simulink model "AFDNFSmodelMPA"  (Simulink 8.8)
settings: Solver=ode45  StartTime=0.0  StopTime=100  FixedStep=1e-3  RelTol=1e-6  EnableMultiTasking=on
InitFcn:
  | run('Methods/AFDSimInit')
  | load('SampleDatcomData.mat')
values from neighbouring files (symbols this model uses):
  nfs = TransferFunction('Plot','true')    [Main.m]    (also in NFSDatabase.sldd = SI
                Imperial
                28184.4409185639)
undefined symbols (not defined in the file or in its folder): datcom, desired, K_lat, K_long, Kobsvlat, Kobsvlong, lat, latsys, long, longsys, Newton, Raphson, sigbuilder_block
libraries: aerolibutil x13, aerolibtransform2 x1, aerolibasang x1
(part 1 of 3)
settings Model: Creator=AHKh PC  LastModifiedBy=AHKh
settings SolverCC: ZeroCrossAlgorithm=Adaptive  AutoInsertRateTranBlk=on
settings DataIOCC: LimitDataPoints=off  SaveOutput=off
settings OptimizationCC: ExpressionDepthLimit=2147483647
settings DebuggingCC: SolverPrmCheckMsg=warning
settings GRTTargetCC: CombineOutputUpdateFcns=on  GRTInterface=off

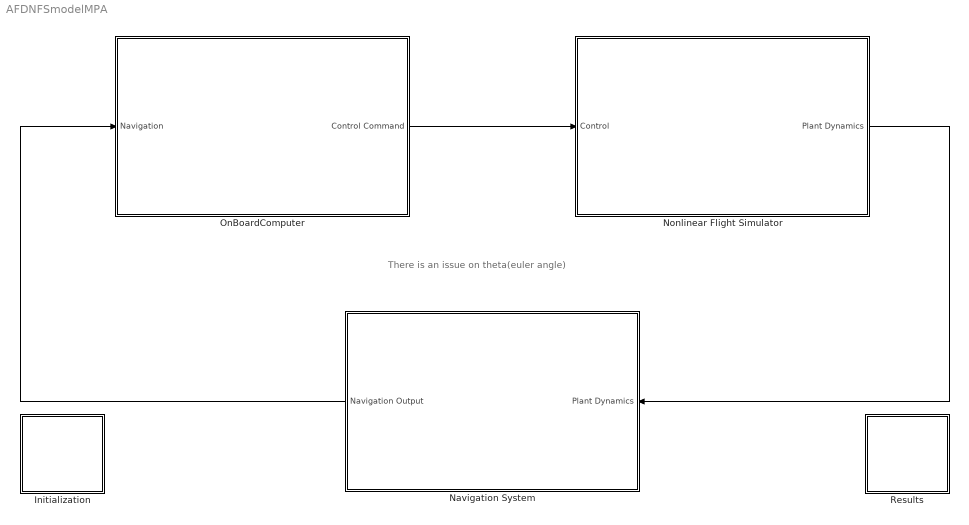
== system AFDNFSmodelMPA ==
  note: There is an issue on theta(euler angle)
  Initialization : Subsystem
      settings: OpenFcn=|
      | % edit('Methods/AFDSimInit.m')
      | !NFSData/NFS Data.xlsx
      mask Display: image(imread('iData/Initialization'))
  Navigation System : Subsystem
      mask Display: image(imread('iData/NavigationSystem'))
  Nonlinear Flight Simulator : Subsystem
      mask Display: image(imread('iData/LockheedMartinVARIOUS'));
  OnBoardComputer : Subsystem
      mask Display: image(imread('iData/OnBoardComputerESAPathfinder'));
  Results : Subsystem
      settings: OpenFcn=|
      | cd 'Methods';
      | Plotter(ned_position,euler_angles,control_commands,tout)
      | cd ..
      mask Display: image(imread('iData/Initialization'))
  wires:
  OnBoardComputer/1(Control Command) -> Nonlinear Flight Simulator/1(Control)
  Navigation System/1(Navigation Output) -> OnBoardComputer/1(Navigation)
  Nonlinear Flight Simulator/1(Plant Dynamics) -> Navigation System/1(Plant Dynamics)

== system AFDNFSmodelMPA/Initialization ==

== system AFDNFSmodelMPA/Navigation System ==
  Plant Dynamics : Inport
  Navigation Output : Outport
  wires:
  Plant Dynamics/1 -> Navigation Output/1

== system AFDNFSmodelMPA/Nonlinear Flight Simulator ==
  Control : Inport
  6DoF Nonlinear Flight Equations of Motion (Rigid Body) : Subsystem
  Forces&Moments : Subsystem
  Ground1 : Ground
  Initialization : Subsystem
  Mux : Mux  Inputs=7
  Plot : Subsystem
  Scope : Scope
  Scope1 : Scope
  Scope4 : Scope
  Plant Dynamics : Outport
  wires:
  Forces&Moments/1(Forces (Body)) -> 6DoF Nonlinear Flight Equations of Motion (Rigid Body)/1(Forces (F) (Body)), Scope1/1
  Forces&Moments/2(Moments (Body)) -> Scope4/1, 6DoF Nonlinear Flight Equations of Motion (Rigid Body)/2(Moments (M) (Body))
  6DoF Nonlinear Flight Equations of Motion (Rigid Body)/1(Linear Velocity (Body)) -> Forces&Moments/1(Linear Velocity), Plot/1(Linear Velocity (Body)), Mux/1
  Initialization/3(Initial Inertia tensor) -> 6DoF Nonlinear Flight Equations of Motion (Rigid Body)/5(Inertia Tensor (I))
  Initialization/4(Inertia tensor Change Rate) -> 6DoF Nonlinear Flight Equations of Motion (Rigid Body)/6(Inertia Tensor Change Rate (Idot))
  Control/1 -> Forces&Moments/3(Control)
  Initialization/2(Mass Consumption Rate) -> 6DoF Nonlinear Flight Equations of Motion (Rigid Body)/4(Mass Consumption Rate)
  Initialization/1(Initial Mass) -> 6DoF Nonlinear Flight Equations of Motion (Rigid Body)/3(Initial Mass)
  Initialization/5(Initial Linear Velocity Vector) -> 6DoF Nonlinear Flight Equations of Motion (Rigid Body)/7(Initial Linear  Velocity Vector)
  Initialization/6(Initial Angular Velocity Vector) -> 6DoF Nonlinear Flight Equations of Motion (Rigid Body)/8(Initial Angular  Velocity Vector)
  Initialization/7(Initial Euler Angles) -> 6DoF Nonlinear Flight Equations of Motion (Rigid Body)/9(Initial Euler Angles)
  6DoF Nonlinear Flight Equations of Motion (Rigid Body)/2(Angular Velocity (Body)) -> Forces&Moments/2(Angular Velocity), Plot/2(Angular Velocity (Body)), Mux/2
  6DoF Nonlinear Flight Equations of Motion (Rigid Body)/4(Angular Acceleration (Body)) -> Plot/4(Angular Acceleration (Body)), Mux/4
  Initialization/8(Initial Location (NED)) -> 6DoF Nonlinear Flight Equations of Motion (Rigid Body)/10(Initial Location (NED))
  6DoF Nonlinear Flight Equations of Motion (Rigid Body)/3(Linear Acceleration (Body)) -> Plot/3(Linear Acceleration (Body)), Mux/3
  6DoF Nonlinear Flight Equations of Motion (Rigid Body)/7(Velocity (NED)) -> Plot/7(Velocity (NED)), Mux/7
  Ground1/1 -> Scope/1
  6DoF Nonlinear Flight Equations of Motion (Rigid Body)/6(Position (NED)) -> Forces&Moments/5(Position), Plot/6(Position (NED)), Mux/6
  6DoF Nonlinear Flight Equations of Motion (Rigid Body)/5(Euler Angles) -> Forces&Moments/4(Attitute), Plot/5(Euler Angles), Mux/5
  Mux/1 -> Plant Dynamics/1

== system AFDNFSmodelMPA/OnBoardComputer ==
  Navigation : Inport
  Control System : Subsystem
  Guidance Algorithm : Subsystem
  Control Command : Outport
  wires:
  Navigation/1 -> Guidance Algorithm/1(Navigation)
  Guidance Algorithm/1(Navigation data & Guidance Command) -> Control System/1(Guidance Command)
  Control System/1(Control Command) -> Control Command/1

== system AFDNFSmodelMPA/Results ==

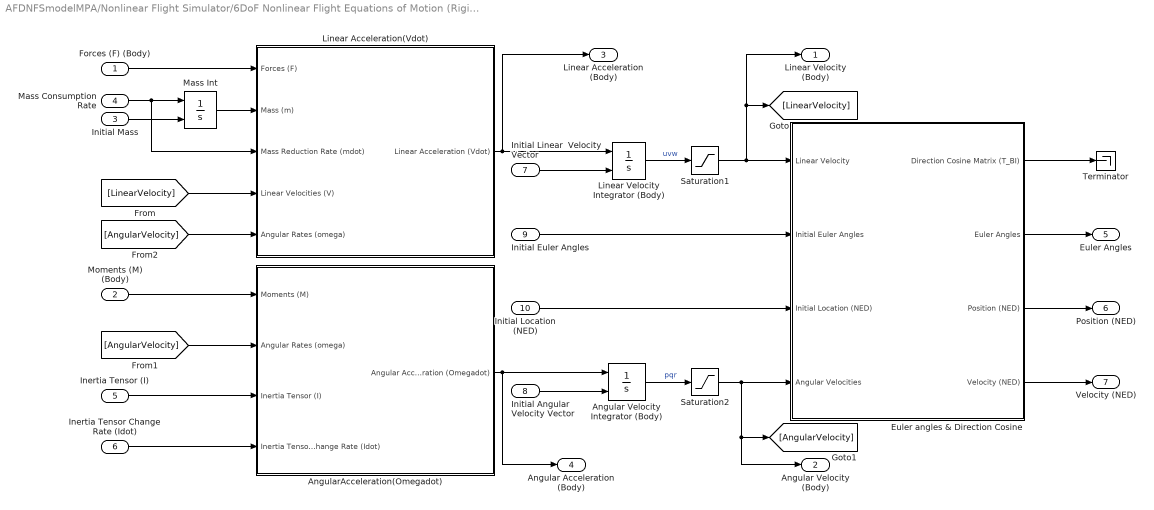
== system AFDNFSmodelMPA/Nonlinear Flight Simulator/6DoF Nonlinear Flight Equations of Motion (Rigid Body) ==
  Forces (F) (Body) : Inport
  Moments (M) (Body) : Inport  Port=2  PortDimensions=[3,1]
  Initial Mass : Inport  Port=3
  Mass Consumption Rate : Inport  Port=4
  Inertia Tensor (I) : Inport  Port=5
  Inertia Tensor Change Rate (Idot) : Inport  Port=6
  Initial Linear  Velocity Vector : Inport  Port=7
  Initial Angular  Velocity Vector : Inport  Port=8
  Initial Euler Angles : Inport  Port=9
  Initial Location (NED) : Inport  Port=10
  Angular Velocity Integrator (Body) : Integrator  InitialConditionSource=external  InitialCondition=nfs.angularvel0
  AngularAcceleration(Omegadot) : Subsystem
  Euler angles & Direction Cosine : Subsystem
  Linear Acceleration(Vdot) : Subsystem
  Linear Velocity Integrator (Body) : Integrator  InitialConditionSource=external  InitialCondition=nfs.crusevelvec  ContinuousStateAttributes='BodyVelocity'
  Mass Int : Integrator  InitialConditionSource=external  InitialCondition=nfs.crusevelvec  ContinuousStateAttributes='BodyVelocity'
  Saturation1 : Saturate  UpperLimit=500  LowerLimit=-500
  Saturation2 : Saturate  UpperLimit=500  LowerLimit=-500
  Terminator : Terminator
  Linear Velocity (Body) : Outport
  Angular Velocity (Body) : Outport  Port=2
  Linear Acceleration (Body) : Outport  Port=3
  Angular Acceleration (Body) : Outport  Port=4
  Euler Angles : Outport  Port=5
  Position (NED) : Outport  Port=6
  Velocity (NED) : Outport  Port=7
  wires:
  Initial Mass/1 -> Mass Int/2
  Mass Int/1 -> Linear Acceleration(Vdot)/2(Mass (m))
  Mass Consumption Rate/1 -> Linear Acceleration(Vdot)/3(Mass Reduction Rate (mdot)), Mass Int/1
  Linear Velocity Integrator (Body)/1 -> Saturation1/1  "uvw"
  Angular Velocity Integrator (Body)/1 -> Saturation2/1  "pqr"
  Inertia Tensor (I)/1 -> AngularAcceleration(Omegadot)/3(Inertia Tensor (I))
  Inertia Tensor Change Rate (Idot)/1 -> AngularAcceleration(Omegadot)/4(Inertia Tensor Change Rate (Idot))
  Euler angles & Direction Cosine/1(Direction Cosine Matrix (T_BI)) -> Terminator/1
  Initial Location (NED)/1 -> Euler angles & Direction Cosine/3(Initial Location (NED))
  Forces (F) (Body)/1 -> Linear Acceleration(Vdot)/1(Forces (F))
  Linear Acceleration(Vdot)/1(Linear Acceleration (Vdot)) -> Linear Acceleration (Body)/1, Linear Velocity Integrator (Body)/1
  Initial Linear  Velocity Vector/1 -> Linear Velocity Integrator (Body)/2
  Initial Angular  Velocity Vector/1 -> Angular Velocity Integrator (Body)/2
  AngularAcceleration(Omegadot)/1(Angular Acceleration (Omegadot)) -> Angular Velocity Integrator (Body)/1, Angular Acceleration (Body)/1
  [LinearVelocity] -> Linear Acceleration(Vdot)/4(Linear Velocities (V))
  [AngularVelocity] -> Linear Acceleration(Vdot)/5(Angular Rates (omega))
  Moments (M) (Body)/1 -> AngularAcceleration(Omegadot)/1(Moments (M))
  [AngularVelocity] -> AngularAcceleration(Omegadot)/2(Angular Rates (omega))
  Initial Euler Angles/1 -> Euler angles & Direction Cosine/2(Initial Euler Angles)
  Euler angles & Direction Cosine/4(Velocity (NED)) -> Velocity (NED)/1
  Euler angles & Direction Cosine/2(Euler Angles) -> Euler Angles/1
  Euler angles & Direction Cosine/3(Position (NED)) -> Position (NED)/1
  Saturation1/1 -> Linear Velocity (Body)/1, [LinearVelocity], Euler angles & Direction Cosine/1(Linear Velocity)
  Saturation2/1 -> Angular Velocity (Body)/1, [AngularVelocity], Euler angles & Direction Cosine/4(Angular Velocities)

== system AFDNFSmodelMPA/Nonlinear Flight Simulator/Forces&Moments ==
  Linear Velocity : Inport
  Angular Velocity : Inport  Port=2  Unit=rad/s  PortDimensions=[3,1]
  Control : Inport  Port=3
  Attitute : Inport  Port=4  PortDimensions=[3,1]
  Position : Inport  Port=5
  Aero Attributes : Subsystem
  Bus Selector : BusSelector  OutputSignals=delta_f,delta_e,delta_a
  C.G Loc : Constant  Value=[0 0 0]'
  Digital DATCOM v1.0.2 : Subsystem  mask(DATCOM Aerodynamic Forces and Moments Estimation){datcom=datcom}
      mask prompts: datcom "Datcom Structure"
      mask Display:
      | port_label('input',1,'\alpha (rad)','texmode','on');
      | port_label('input',2,'\beta (rad)','texmode','on');
      | port_label('input',3,'Mach','texmode','on');
      | port_label('input',4,'h (m)','texmode','on');
      | port_label('input',5,'q_{bar}','texmode','on');
      | port_label('input',6,'d\alpha/dt (rad/s)','texmode','on');
      | port_label('input',7,'V_{body} m/s','texmode','on');
      | port_label('input',8,'\omega (rad/s)','texmode','on');
      | port_label('input',9,'\delta_F (rad)','texmode','on');
      | port_label('input',10,'\delta_E (rad)','texmode','on');
      | port_label('input',11,'\delta_A (rad)','texmode','on');
      | port_label('input',12,'C.G. (m)','texmode','on');
      | port_label('output',1,'F_{body} (N)','texmode','on');
      | port_label('output',2,'M_{body} (N.m)','texmode','on');
  HeightInENU : Gain  Gain=-1  SaturateOnIntegerOverflow=on  OutDataTypeStr=Inherit: Same as input  ParamDataTypeStr=Inherit: Same as input
  HeightInENU1 : Gain  Gain=-1  SaturateOnIntegerOverflow=on  OutDataTypeStr=Inherit: Same as input  ParamDataTypeStr=Inherit: Same as input
  Linear Velocity 1 : InportShadow
  Position 1 : InportShadow  Port=5
  Selector : Selector  InputPortWidth=3  IndexOptions=Index vector (dialog)  Indices=[3]  OutputSizes=1
  Selector1 : Selector  InputPortWidth=3  IndexOptions=Index vector (dialog)  Indices=[3]  OutputSizes=1
  Sum : Sum  Inputs=+++
  Sum1 : Sum  Inputs=+++
  Terminator1 : Terminator
  Thrust : Subsystem
  Weight : Subsystem
  Forces (Body) : Outport
  Moments (Body) : Outport  Port=2
  wires:
  HeightInENU/1 -> Aero Attributes/2(Altitude)
  Linear Velocity/1 -> Aero Attributes/1(Linear Velocity (Body))
  Aero Attributes/4(Betadot) -> Terminator1/1
  Angular Velocity/1 -> Digital DATCOM v1.0.2/8(p,q,r)
  Selector/1 -> HeightInENU1/1
  Position/1 -> Selector/1
  Position 1/1 -> Selector1/1
  HeightInENU1/1 -> Digital DATCOM v1.0.2/4(altitude)
  Selector1/1 -> HeightInENU/1
  Control/1 -> Bus Selector/1
  Bus Selector/1 -> Digital DATCOM v1.0.2/9(delta_f)  "<delta_f>"
  Bus Selector/2 -> Digital DATCOM v1.0.2/10(delta_e)  "<delta_e>"
  Bus Selector/3 -> Digital DATCOM v1.0.2/11(delta_a)  "<delta_a>"
  Linear Velocity 1/1 -> Digital DATCOM v1.0.2/7(V)
  Aero Attributes/1(Alpha) -> Digital DATCOM v1.0.2/1(alp ha)
  Aero Attributes/2(Beta) -> Digital DATCOM v1.0.2/2(beta)
  Aero Attributes/5(Dynamic Pressure) -> Digital DATCOM v1.0.2/5(qbar)
  Aero Attributes/3(Mach) -> Digital DATCOM v1.0.2/3(Mach)
  Aero Attributes/6(Alphadot) -> Digital DATCOM v1.0.2/6(alpha_dot)
  Attitute/1 -> Weight/1(Attitute)
  Digital DATCOM v1.0.2/1(F) -> Sum/1
  Weight/1(Force) -> Sum/2
  Thrust/1(Force) -> Sum/3
  Sum/1 -> Forces (Body)/1
  Weight/2(Moment) -> Sum1/2
  Digital DATCOM v1.0.2/2(M) -> Sum1/1
  Thrust/2(Moment) -> Sum1/3
  Sum1/1 -> Moments (Body)/1
  C.G Loc/1 -> Digital DATCOM v1.0.2/12(C.G.)

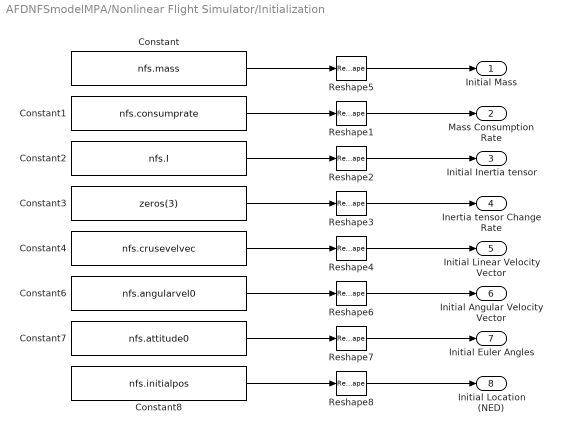
== system AFDNFSmodelMPA/Nonlinear Flight Simulator/Initialization ==
  Constant : Constant  Value=nfs.mass
  Constant1 : Constant  Value=nfs.consumprate
  Constant2 : Constant  Value=nfs.I
  Constant3 : Constant  Value=zeros(3)
  Constant4 : Constant  Value=nfs.crusevelvec
  Constant6 : Constant  Value=nfs.angularvel0
  Constant7 : Constant  Value=nfs.attitude0
  Constant8 : Constant  Value=nfs.initialpos
  Reshape1 : Reshape
  Reshape2 : Reshape  OutputDimensionality=Customize  OutputDimensions=[3,3]
  Reshape3 : Reshape  OutputDimensionality=Customize  OutputDimensions=[3,3]
  Reshape{4,6..8} (4 alike) : Reshape  OutputDimensionality=Column vector (2-D)
  Reshape5 : Reshape
  Initial Mass : Outport
  Mass Consumption Rate : Outport  Port=2
  Initial Inertia tensor : Outport  Port=3
  Inertia tensor Change Rate : Outport  Port=4
  Initial Linear Velocity Vector : Outport  Port=5
  Initial Angular Velocity Vector : Outport  Port=6
  Initial Euler Angles : Outport  Port=7
  Initial Location (NED) : Outport  Port=8
  wires:
  Constant/1 -> Reshape5/1
  Constant1/1 -> Reshape1/1
  Constant2/1 -> Reshape2/1
  Constant3/1 -> Reshape3/1
  Constant4/1 -> Reshape4/1
  Constant6/1 -> Reshape6/1
  Constant7/1 -> Reshape7/1
  Constant8/1 -> Reshape8/1
  Reshape5/1 -> Initial Mass/1
  Reshape1/1 -> Mass Consumption Rate/1
  Reshape2/1 -> Initial Inertia tensor/1
  Reshape3/1 -> Inertia tensor Change Rate/1
  Reshape4/1 -> Initial Linear Velocity Vector/1
  Reshape6/1 -> Initial Angular Velocity Vector/1
  Reshape7/1 -> Initial Euler Angles/1
  Reshape8/1 -> Initial Location (NED)/1

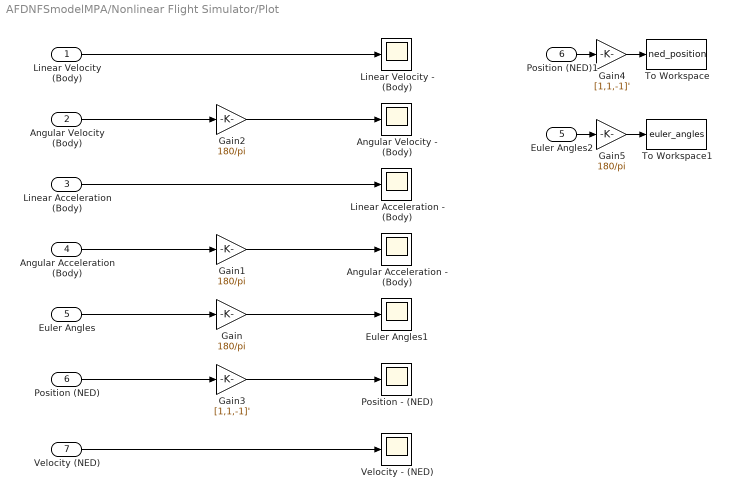
== system AFDNFSmodelMPA/Nonlinear Flight Simulator/Plot ==
  Linear Velocity (Body) : Inport
  Angular Velocity (Body) : Inport  Port=2
  Linear Acceleration (Body) : Inport  Port=3
  Angular Acceleration (Body) : Inport  Port=4
  Euler Angles : Inport  Port=5  PortDimensions=3
  Position (NED) : Inport  Port=6  PortDimensions=3
  Velocity (NED) : Inport  Port=7
  Angular Acceleration - (Body) : Scope
  Angular Velocity - (Body) : Scope
  Euler Angles1 : Scope
  Euler Angles2 : InportShadow  Port=5  PortDimensions=3
  Gain{,1..2,5} (4 alike) : Gain  Gain=180/pi
  Gain3 : Gain  Gain=[1,1,-1]'
  Gain4 : Gain  Gain=[1,1,-1]'
  Linear Acceleration - (Body) : Scope
  Linear Velocity - (Body) : Scope
  Position (NED)1 : InportShadow  Port=6  PortDimensions=3
  Position - (NED) : Scope
  To Workspace : ToWorkspace  VariableName=ned_position  SampleTime=-1
  To Workspace1 : ToWorkspace  VariableName=euler_angles  SampleTime=-1
  Velocity - (NED) : Scope
  wires:
  Gain/1 -> Euler Angles1/1
  Euler Angles/1 -> Gain/1
  Position (NED)/1 -> Gain3/1
  Linear Velocity (Body)/1 -> Linear Velocity - (Body)/1
  Angular Velocity (Body)/1 -> Gain2/1
  Linear Acceleration (Body)/1 -> Linear Acceleration - (Body)/1
  Angular Acceleration (Body)/1 -> Gain1/1
  Velocity (NED)/1 -> Velocity - (NED)/1
  Gain1/1 -> Angular Acceleration - (Body)/1
  Gain2/1 -> Angular Velocity - (Body)/1
  Gain3/1 -> Position - (NED)/1
  Position (NED)1/1 -> Gain4/1
  Gain4/1 -> To Workspace/1
  Euler Angles2/1 -> Gain5/1
  Gain5/1 -> To Workspace1/1

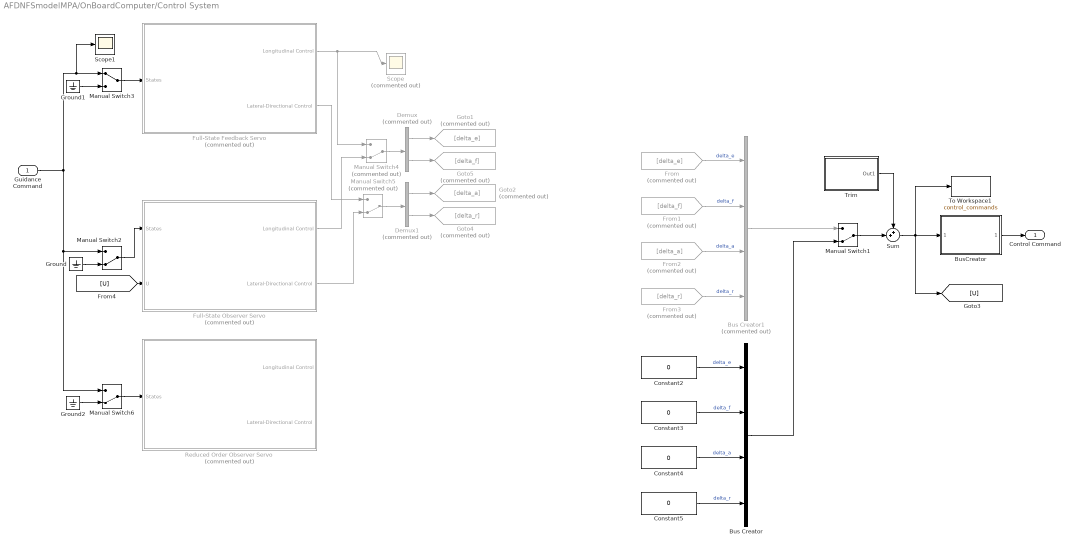
== system AFDNFSmodelMPA/OnBoardComputer/Control System ==
  Guidance Command : Inport
  Bus Creator : BusCreator  Inputs=4
  Bus Creator1 : BusCreator  Commented=on  Inputs=4
  BusCreator : Subsystem
  Constant{2..5} (4 alike) : Constant  Value=0
  Demux : Demux  Commented=on  Outputs=2
  Demux1 : Demux  Commented=on  Outputs=2
  From : From  Commented=on  GotoTag=delta_e
  From1 : From  Commented=on  GotoTag=delta_f
  From2 : From  Commented=on  GotoTag=delta_a
  From3 : From  Commented=on  GotoTag=delta_r
  Full-State Feedback Servo : Subsystem  Commented=on
  Full-State Observer Servo : Subsystem  Commented=on
  Goto1 : Goto  Commented=on  GotoTag=delta_e
  Goto2 : Goto  Commented=on  GotoTag=delta_a
  Goto4 : Goto  Commented=on  GotoTag=delta_r
  Goto5 : Goto  Commented=on  GotoTag=delta_f
  Ground : Ground
  Ground1 : Ground
  Ground2 : Ground
  Manual Switch1 : ManualSwitch  CurrentSetting=0
  Manual Switch2 : ManualSwitch  CurrentSetting=0
  Manual Switch3 : ManualSwitch
  Manual Switch4 : ManualSwitch  Commented=on  CurrentSetting=0
  Manual Switch5 : ManualSwitch  Commented=on  CurrentSetting=0
  Manual Switch6 : ManualSwitch  CurrentSetting=0
  Reduced Order Observer Servo : Subsystem  Commented=on
  Scope : Scope  Commented=on
  Scope1 : Scope
  Sum : Sum  Inputs=++|
  To Workspace1 : ToWorkspace  VariableName=control_commands  SampleTime=-1
  Trim : Subsystem
  Control Command : Outport
  wires:
  Trim/1(Out1) -> Sum/1
  Bus Creator/1 -> Manual Switch1/2
  Manual Switch1/1 -> Sum/2
  Demux/1 -> Goto1/1
  Demux/2 -> Goto5/1
  Demux1/1 -> Goto2/1
  Demux1/2 -> Goto4/1
  Manual Switch2/1 -> Full-State Observer Servo/1(States)
  Manual Switch3/1 -> Full-State Feedback Servo/1(States)
  Ground/1 -> Manual Switch2/2
  Ground1/1 -> Manual Switch3/2
  Guidance Command/1 -> Manual Switch2/1, Manual Switch6/1, Manual Switch3/1, Scope1/1
  Full-State Feedback Servo/1(Longitudinal Control) -> Manual Switch4/1, Scope/1
  Full-State Feedback Servo/2(Lateral-Directional Control) -> Manual Switch5/1
  Full-State Observer Servo/1(Longitudinal Control) -> Manual Switch4/2
  Full-State Observer Servo/2(Lateral-Directional Control) -> Manual Switch5/2
  Manual Switch4/1 -> Demux/1
  Manual Switch5/1 -> Demux1/1
  Ground2/1 -> Manual Switch6/2
  Manual Switch6/1 -> Reduced Order Observer Servo/1(States)
  [U] -> Full-State Observer Servo/2(U)
  Constant2/1 -> Bus Creator/1  "delta_e"
  Constant3/1 -> Bus Creator/2  "delta_f"
  Constant5/1 -> Bus Creator/4  "delta_r"
  Constant4/1 -> Bus Creator/3  "delta_a"
  Bus Creator1/1 -> Manual Switch1/1
  From/1 -> Bus Creator1/1  "delta_e"
  From1/1 -> Bus Creator1/2  "delta_f"
  From3/1 -> Bus Creator1/4  "delta_r"
  From2/1 -> Bus Creator1/3  "delta_a"
  Sum/1 -> BusCreator/1(" "), To Workspace1/1, [U]
  BusCreator/1("  ") -> Control Command/1

== system AFDNFSmodelMPA/OnBoardComputer/Guidance Algorithm ==
  note: There is no guidance algorithm yet!
  Navigation : Inport
  Constant : Constant  Value=desired.pitch
  Constant1 : Constant  Value=[nfs.crusevelvec(1); nfs.crusevelvec(3)]
  Constant2 : Constant  Value=nfs.crusevelvec(2)
  Demux : Demux  Outputs=7
  Mux : Mux  Inputs=2
  Mux1 : Mux  Inputs=3
  Mux2 : Mux  Inputs=3
  Selector : Selector  InputPortWidth=3  IndexOptions=Index vector (dialog)  Indices=[2]  OutputSizes=1
  Selector1 : Selector  InputPortWidth=3  IndexOptions=Index vector (dialog)  Indices=[2]  OutputSizes=1
  Selector2 : Selector  InputPortWidth=3  IndexOptions=Index vector (dialog)  Indices=[2]  OutputSizes=1
  Selector3 : Selector  InputPortWidth=3  IndexOptions=Index vector (dialog)  Indices=[1 3]  OutputSizes=1
  Selector4 : Selector  InputPortWidth=3  IndexOptions=Index vector (dialog)  Indices=[1 3]  OutputSizes=1
  Selector5 : Selector  InputPortWidth=3  IndexOptions=Index vector (dialog)  Indices=[1 3]  OutputSizes=1
  Sum : Sum  Inputs=|+-
  Sum1 : Sum  Inputs=-+|
  Sum2 : Sum  Inputs=|+-
  Terminator{1..4} (4 alike) : Terminator
  Navigation data & Guidance Command : Outport
  wires:
  Navigation/1 -> Demux/1
  Demux/1 -> Selector3/1, Selector1/1  "Linear Velocity (Body)"
  Demux/3 -> Terminator1/1  "Linear Acceleration (Body)"
  Demux/4 -> Terminator2/1  "Angular Acceleration (Body)"
  Demux/7 -> Terminator4/1  "Velocity (NED)"
  Demux/2 -> Selector/1, Selector4/1  "Angular Velocity (Body)"
  Demux/6 -> Terminator3/1  "Position (NED)"
  Demux/5 -> Selector2/1, Selector5/1  "Euler Angles"
  Mux/1 -> Navigation data & Guidance Command/1
  Mux1/1 -> Mux/1
  Mux2/1 -> Mux/2
  Selector/1 -> Mux1/2  "q"
  Selector4/1 -> Mux2/2  "p & r"
  Selector5/1 -> Mux2/3  "phi & psi"
  Selector2/1 -> Sum/1  "Theta"
  Sum/1 -> Mux1/3
  Constant/1 -> Sum/2
  Sum1/1 -> Mux1/1
  Selector3/1 -> Sum1/2  "u & w"
  Constant1/1 -> Sum1/1
  Selector1/1 -> Sum2/1  "v"
  Sum2/1 -> Mux2/1
  Constant2/1 -> Sum2/2

== system AFDNFSmodelMPA/Nonlinear Flight Simulator/6DoF Nonlinear Flight Equations of Motion (Rigid Body)/AngularAcceleration(Omegadot) ==
  Moments (M) : Inport  PortDimensions=[3,1]
  Angular Rates (omega) : Inport  Port=2  PortDimensions=[3,1]
  Inertia Tensor (I) : Inport  Port=3
  Inertia Tensor Change Rate (Idot) : Inport  Port=4
  Angular Rates (omega)1 : InportShadow  Port=2  PortDimensions=[3,1]
  Cross Product : Subsystem  mask(Cross Product){}
      mask help: Calculate the cross product of two 3-by-1 vectors.
      mask Display:
      | text(.5,.5,'Cross\nProduct\nC = AxB', ...
      | 	'HorizontalAlignment','Center',...
      | 	'VerticalAlignment','middle')
  Inertia Tensor (I)1 : InportShadow  Port=3
  Product1 : Product  Inputs=**  Multiplication=Matrix(*)  SaturateOnIntegerOverflow=on  OutDataTypeStr=Inherit: Same as first input
  Product3 : Product  Inputs=**  Multiplication=Matrix(*)  SaturateOnIntegerOverflow=on  OutDataTypeStr=Inherit: Same as first input
  Product4 : Product  Inputs=/*  Multiplication=Matrix(*)  SaturateOnIntegerOverflow=on  OutDataTypeStr=Inherit: Same as first input
  Sum1 : Sum  Inputs=|+-  SaturateOnIntegerOverflow=on
  Sum3 : Sum  Inputs=|+-  SaturateOnIntegerOverflow=on
  Angular Acceleration (Omegadot) : Outport
  wires:
  Product3/1 -> Sum1/2
  Product1/1 -> Cross Product/2(B)
  Cross Product/1(C) -> Sum3/2
  Sum1/1 -> Sum3/1
  Sum3/1 -> Product4/2
  Product4/1 -> Angular Acceleration (Omegadot)/1
  Inertia Tensor (I)1/1 -> Product4/1
  Moments (M)/1 -> Sum1/1
  Inertia Tensor Change Rate (Idot)/1 -> Product3/1
  Angular Rates (omega)/1 -> Cross Product/1(A), Product3/2
  Angular Rates (omega)1/1 -> Product1/2
  Inertia Tensor (I)/1 -> Product1/1

== system AFDNFSmodelMPA/Nonlinear Flight Simulator/6DoF Nonlinear Flight Equations of Motion (Rigid Body)/Euler angles & Direction Cosine ==
  Linear Velocity : Inport  PortDimensions=[3,1]
  Initial Euler Angles : Inport  Port=2
  Initial Location (NED) : Inport  Port=3  PortDimensions=[3,1]
  Angular Velocities : Inport  Port=4
  Constant : Constant
  Euler Angles Int : Integrator  InitialConditionSource=external  InitialCondition=nfs.attitude0
  Euler angles Calculation : Subsystem
  If : If  IfExpression=u1(3)>= 0  ShowElse=off
  If Action Subsystem : Subsystem  TreatAsAtomicUnit=on
  Position Integrator : Integrator  InitialConditionSource=external  InitialCondition=[0,0,nfs.attitude0]
  Rotation Angles to DCM : Subsystem
  Selector : Selector  InputPortWidth=3  IndexOptions=Index vector (dialog)  Indices=[3 2 1]  OutputSizes=1
  Transform from Body to Inertial axes : Subsystem
      mask Display: disp('T_IB')
  Transpose : Math  Operator=transpose  SaturateOnIntegerOverflow=on
  Direction Cosine Matrix (T_BI) : Outport  PortDimensions=[3,3]
  Euler Angles : Outport  Port=2
  Position (NED) : Outport  Port=3  PortDimensions=[3,1]
  Velocity (NED) : Outport  Port=4  PortDimensions=[3,1]
  wires:
  Initial Euler Angles/1 -> Euler Angles Int/2
  Rotation Angles to DCM/1(DCM) -> Transpose/1, Direction Cosine Matrix (T_BI)/1
  Angular Velocities/1 -> Euler angles Calculation/1(Angular Velocities)
  Selector/1 -> Rotation Angles to DCM/1("[R1,R2,R3]")
  Transpose/1 -> Transform from Body to Inertial axes/1(Transformation Matrix)
  Linear Velocity/1 -> Transform from Body to Inertial axes/2(Position Vector)
  Initial Location (NED)/1 -> Position Integrator/2
  Euler Angles Int/1 -> Euler Angles/1, Selector/1, Euler angles Calculation/2(Euler Angles)
  Transform from Body to Inertial axes/1(Ve) -> Velocity (NED)/1, Position Integrator/1
  Position Integrator/1 -> Position (NED)/1, If/1
  Euler angles Calculation/1(Euler Rates) -> Euler Angles Int/1
  If/1 -> If Action Subsystem/Action
  Constant/1 -> If Action Subsystem/1(Simulation Termination)

== system AFDNFSmodelMPA/Nonlinear Flight Simulator/6DoF Nonlinear Flight Equations of Motion (Rigid Body)/Linear Acceleration(Vdot) ==
  Forces (F) : Inport  PortDimensions=[3,1]
  Mass (m) : Inport  Port=2
  Mass Reduction Rate (mdot) : Inport  Port=3
  Linear Velocities (V) : Inport  Port=4  PortDimensions=[3,1]
  Angular Rates (omega) : Inport  Port=5
  Cross Product : Subsystem  mask(Cross Product){}
      mask help: Calculate the cross product of two 3-by-1 vectors.
      mask Display:
      | text(.5,.5,'Cross\nProduct\nC = AxB', ...
      | 	'HorizontalAlignment','Center',...
      | 	'VerticalAlignment','middle')
  Linear Velocities (V)1 : InportShadow  Port=4  PortDimensions=[3,1]
  Mass (m)1 : InportShadow  Port=2
  Product : Product  Inputs=*/  SaturateOnIntegerOverflow=on  OutDataTypeStr=Inherit: Same as first input
  Product1 : Product  Inputs=*/  SaturateOnIntegerOverflow=on  OutDataTypeStr=Inherit: Same as first input
  Product3 : Product  Inputs=**  SaturateOnIntegerOverflow=on  OutDataTypeStr=Inherit: Same as first input
  Sum1 : Sum  Inputs=|+-  SaturateOnIntegerOverflow=on
  Sum3 : Sum  Inputs=|+-  SaturateOnIntegerOverflow=on
  Linear Acceleration (Vdot) : Outport
  wires:
  Mass (m)/1 -> Product/2
  Product/1 -> Sum1/1
  Mass Reduction Rate (mdot)/1 -> Product1/1
  Mass (m)1/1 -> Product1/2
  Product1/1 -> Product3/1
  Product3/1 -> Sum1/2
  Sum1/1 -> Sum3/1
  Cross Product/1(C) -> Sum3/2
  Linear Velocities (V)/1 -> Product3/2
  Forces (F)/1 -> Product/1
  Sum3/1 -> Linear Acceleration (Vdot)/1
  Angular Rates (omega)/1 -> Cross Product/1(A)
  Linear Velocities (V)1/1 -> Cross Product/2(B)

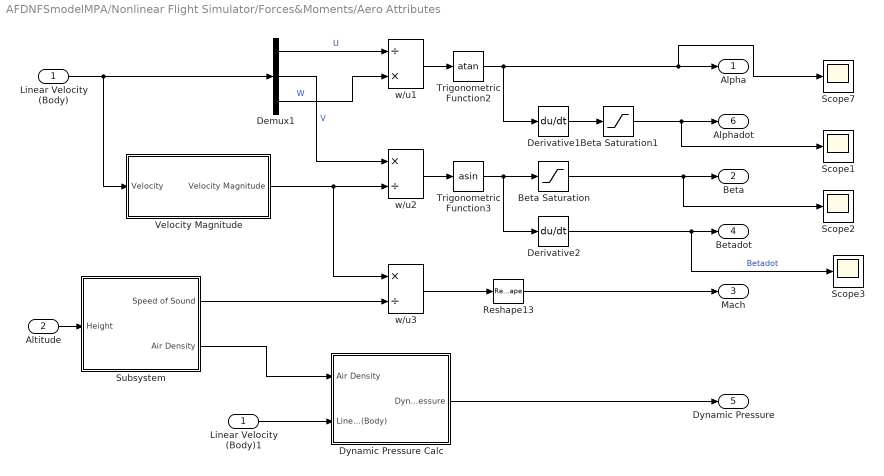
== system AFDNFSmodelMPA/Nonlinear Flight Simulator/Forces&Moments/Aero Attributes ==
  Linear Velocity (Body) : Inport  PortDimensions=[3,1]
  Altitude : Inport  Port=2
  Beta Saturation : Saturate  UpperLimit=5*pi/11  LowerLimit=-5*pi/11
  Beta Saturation1 : Saturate  UpperLimit=1  LowerLimit=-1
  Demux1 : Demux  Outputs=3
  Derivative1 : Derivative
  Derivative2 : Derivative
  Dynamic Pressure Calc : Subsystem
  Linear Velocity (Body)1 : InportShadow  PortDimensions=[3,1]
  Reshape13 : Reshape
  Scope{1..3,7} (4 alike) : Scope
  Subsystem : Subsystem
  Trigonometric Function2 : Trigonometry  Operator=atan
  Trigonometric Function3 : Trigonometry  Operator=asin
  Velocity Magnitude : Subsystem
  w/u1 : Product  Inputs=/*  SaturateOnIntegerOverflow=on  InputSameDT=on  OutDataTypeStr=Inherit: Same as first input
  w/u2 : Product  Inputs=*/  SaturateOnIntegerOverflow=on  InputSameDT=on  OutDataTypeStr=Inherit: Same as first input
  w/u3 : Product  Inputs=*/  SaturateOnIntegerOverflow=on  InputSameDT=on  OutDataTypeStr=Inherit: Same as first input
  Alpha : Outport
  Beta : Outport  Port=2
  Mach : Outport  Port=3
  Betadot : Outport  Port=4
  Dynamic Pressure : Outport  Port=5
  Alphadot : Outport  Port=6
  wires:
  Beta Saturation1/1 -> Alphadot/1, Scope1/1
  Subsystem/2(Air Density) -> Dynamic Pressure Calc/1(Air Density)
  Subsystem/1(Speed of Sound) -> w/u3/2
  Velocity Magnitude/1(Velocity Magnitude) -> w/u3/1, w/u2/2
  Reshape13/1 -> Mach/1
  Derivative2/1 -> Betadot/1, Scope3/1  "Betadot"
  Beta Saturation/1 -> Beta/1, Scope2/1
  Derivative1/1 -> Beta Saturation1/1
  Dynamic Pressure Calc/1(Dynamic Pressure) -> Dynamic Pressure/1
  Linear Velocity (Body)1/1 -> Dynamic Pressure Calc/2(Linear Velocity (Body))
  Altitude/1 -> Subsystem/1(Height)
  w/u3/1 -> Reshape13/1
  Trigonometric Function3/1 -> Beta Saturation/1, Derivative2/1
  Trigonometric Function2/1 -> Derivative1/1, Alpha/1, Scope7/1
  w/u2/1 -> Trigonometric Function3/1
  w/u1/1 -> Trigonometric Function2/1
  Demux1/3 -> w/u1/2  "W"
  Demux1/2 -> w/u2/1  "V"
  Demux1/1 -> w/u1/1  "U"
  Linear Velocity (Body)/1 -> Velocity Magnitude/1(Velocity), Demux1/1

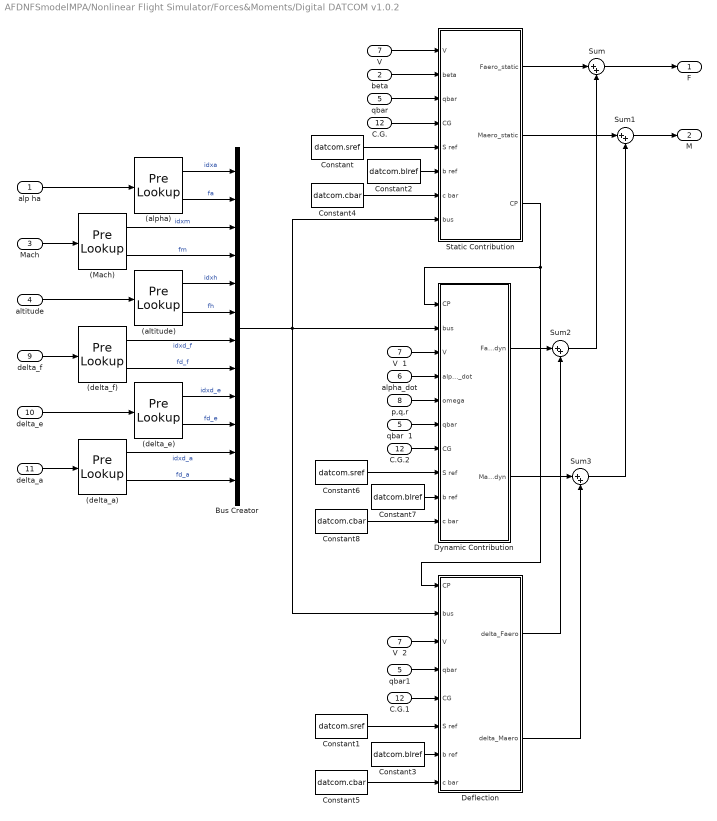
== system AFDNFSmodelMPA/Nonlinear Flight Simulator/Forces&Moments/Digital DATCOM v1.0.2 ==
  alp ha : Inport  Unit=rad
  beta : Inport  Port=2  Unit=rad
  Mach : Inport  Port=3  Unit=1
  altitude : Inport  Port=4  Unit=m
  qbar : Inport  Port=5  Unit=Pa
  alpha_dot : Inport  Port=6  Unit=rad/s
  V : Inport  Port=7  Unit=m/s
  p,q,r : Inport  Port=8  Unit=rad/s
  delta_f : Inport  Port=9  Unit=rad
  delta_e : Inport  Port=10  Unit=rad
  delta_a : Inport  Port=11  Unit=rad
  C.G. : Inport  Port=12  Unit=m
  (Mach) : PreLookup  BreakpointsData=datcom.mach  BeginIndexSearchUsingPreviousIndexResult=on  IndexDataTypeStr=int32  FractionDataTypeStr=double
  (alpha) : PreLookup  BreakpointsData=datcom.alpha  BeginIndexSearchUsingPreviousIndexResult=on  IndexDataTypeStr=int32  FractionDataTypeStr=double
  (altitude) : PreLookup  BreakpointsData=datcom.alt  BeginIndexSearchUsingPreviousIndexResult=on  IndexDataTypeStr=int32  FractionDataTypeStr=double
  (delta_a) : PreLookup  BreakpointsData=datcom.deltal-datcom.deltar  BeginIndexSearchUsingPreviousIndexResult=on  IndexDataTypeStr=int32  FractionDataTypeStr=double
  (delta_e) : PreLookup  BreakpointsData=datcom.delta  BeginIndexSearchUsingPreviousIndexResult=on  IndexDataTypeStr=int32  FractionDataTypeStr=double
  (delta_f) : PreLookup  BreakpointsData=datcom.delta  BeginIndexSearchUsingPreviousIndexResult=on  IndexDataTypeStr=int32  FractionDataTypeStr=double
  Bus Creator : BusCreator  Inputs=12
  C.G.1 : InportShadow  Port=12  Unit=m
  C.G.2 : InportShadow  Port=12  Unit=m
  Constant : Constant  Value=datcom.sref
  Constant1 : Constant  Value=datcom.sref
  Constant2 : Constant  Value=datcom.blref
  Constant3 : Constant  Value=datcom.blref
  Constant4 : Constant  Value=datcom.cbar
  Constant5 : Constant  Value=datcom.cbar
  Constant6 : Constant  Value=datcom.sref
  Constant7 : Constant  Value=datcom.blref
  Constant8 : Constant  Value=datcom.cbar
  Deflection : Subsystem
  Dynamic Contribution : Subsystem
  Static Contribution : Subsystem
  Sum{,1..3} (4 alike) : Sum  Inputs=|++
  V  1 : InportShadow  Port=7  Unit=m/s
  V  2 : InportShadow  Port=7  Unit=m/s
  qbar  1 : InportShadow  Port=5  Unit=Pa
  qbar1 : InportShadow  Port=5  Unit=Pa
  F : Outport  Unit=N
  M : Outport  Port=2  Unit=N*m
  wires:
  Constant8/1 -> Dynamic Contribution/10(c bar)
  Constant6/1 -> Dynamic Contribution/8(S ref)
  Constant7/1 -> Dynamic Contribution/9(b ref)
  C.G.2/1 -> Dynamic Contribution/7(CG)
  Constant4/1 -> Static Contribution/7(c bar)
  Constant5/1 -> Deflection/8(c bar)
  Constant3/1 -> Deflection/7(b ref)
  Constant2/1 -> Static Contribution/6(b ref)
  Constant1/1 -> Deflection/6(S ref)
  Constant/1 -> Static Contribution/5(S ref)
  C.G.1/1 -> Deflection/5(CG)
  C.G./1 -> Static Contribution/4(CG)
  Deflection/2(delta_Maero) -> Sum3/2
  Deflection/1(delta_Faero) -> Sum2/2
  Sum3/1 -> Sum1/2
  Sum2/1 -> Sum/2
  qbar1/1 -> Deflection/4(qbar)
  V  2/1 -> Deflection/3("V ")
  (delta_a)/2 -> Bus Creator/12  "fd_a"
  (delta_a)/1 -> Bus Creator/11  "idxd_a"
  delta_a/1 -> (delta_a)/1
  (delta_e)/2 -> Bus Creator/10  "fd_e"
  (delta_e)/1 -> Bus Creator/9  "idxd_e"
  delta_e/1 -> (delta_e)/1
  V/1 -> Static Contribution/1("V ")
  V  1/1 -> Dynamic Contribution/3(V)
  qbar/1 -> Static Contribution/3(qbar)
  beta/1 -> Static Contribution/2(beta)
  alp ha/1 -> (alpha)/1
  (alpha)/2 -> Bus Creator/2  "fa"
  (Mach)/2 -> Bus Creator/4  "fm"
  (altitude)/2 -> Bus Creator/6  "fh"
  (altitude)/1 -> Bus Creator/5  "idxh"
  (delta_f)/2 -> Bus Creator/8  "fd_f"
  (delta_f)/1 -> Bus Creator/7  "idxd_f"
  altitude/1 -> (altitude)/1
  qbar  1/1 -> Dynamic Contribution/6(qbar)
  p,q,r/1 -> Dynamic Contribution/5(omega)
  alpha_dot/1 -> Dynamic Contribution/4(alpha_dot)
  Sum1/1 -> M/1
  Sum/1 -> F/1
  Dynamic Contribution/2(Maero_dyn) -> Sum3/1
  Static Contribution/2(Maero_static) -> Sum1/1
  Dynamic Contribution/1(Faero_dyn) -> Sum2/1
  Static Contribution/1(Faero_static) -> Sum/1
  Static Contribution/3("CP ") -> Deflection/1(CP), Dynamic Contribution/1(CP)
  Mach/1 -> (Mach)/1
  (Mach)/1 -> Bus Creator/3  "idxm"
  (alpha)/1 -> Bus Creator/1  "idxa"
  delta_f/1 -> (delta_f)/1
  Bus Creator/1 -> Deflection/2(bus), Dynamic Contribution/2(bus), Static Contribution/8(bus)

== system AFDNFSmodelMPA/Nonlinear Flight Simulator/Forces&Moments/Thrust ==
  Manual Switch : ManualSwitch  CurrentSetting=0
  Mux1 : Mux  Inputs=3
  Product : Product  RndMeth=Zero
  Signal Builder : Subsystem  Tag=STV Subsys  LoadFcn=sigbuilder_block('load');  StartFcn=sigbuilder_block('start');  StopFcn=sigbuilder_block('stop');  ClipboardFcn=sigbuilder_block('clipboard');  mask(Sigbuilder block){tuvar=[0:10]}
      mask help: Simulink:masks:SigbuilderBlock_MD
      mask init:
      | if ~strcmp(get_param(bdroot(gcbh),'SimulationStatus'),'stopped') tuvar = sigbuilder_block('maskInit'); end
      settings: CopyFcn=sigbuilder_block('copy');  DeleteFcn=sigbuilder_block('delete');  ModelCloseFcn=sigbuilder_block('modelClose');  PreSaveFcn=sigbuilder_block('preSave');  PauseFcn=sigbuilder_block('pause');  ContinueFcn=sigbuilder_block('continue');  NameChangeFcn=sigbuilder_block('namechange');  OpenFcn=sigbuilder_block('open',[437.25 199.5 550.5 399.75 ]);  CloseFcn=sigbuilder_block('close');
      mask Display: plot(0, 0, 100, 100,[2, 2, 32, 32, 2], [68, 8, 8, 68, 68],[32, 2], [38, 38], [32, 19, 2],[53, 60, 44], [32, 17, 17, 2],[16, 16, 31, 31]);txt = getActiveGroup(gcbh);text(2, 100, txt,'verticalAlignment', 'top');
  Throttle : Gain
  Trim Thrust1 : Constant  Value=nfs.trim.thrust*cos(nfs.tmisalign)
  Trim Thrust2 : Constant  Value=nfs.trim.thrust*sin(nfs.tmisalign)
  Trim Thrust3 : Constant  Value=0
  Trim Thrust4 : Constant
  Trim Thrust5 : Constant  Value=[0 0 0]'
  Force : Outport  Unit=N  PortDimensions=[3,1]
  Moment : Outport  Port=2  Unit=N*m  PortDimensions=[3,1]
  wires:
  Mux1/1 -> Throttle/1
  Trim Thrust3/1 -> Mux1/3
  Trim Thrust2/1 -> Mux1/2
  Trim Thrust1/1 -> Mux1/1
  Throttle/1 -> Product/1
  Product/1 -> Force/1
  Manual Switch/1 -> Product/2
  Signal Builder/1(ThrustDeviation) -> Manual Switch/1
  Trim Thrust4/1 -> Manual Switch/2
  Trim Thrust5/1 -> Moment/1

== system AFDNFSmodelMPA/Nonlinear Flight Simulator/Forces&Moments/Weight ==
  note: theta
  note: phi
  Attitute : Inport  PortDimensions=[3,1]
  Demux : Demux  Outputs=3
  Gain1 : Gain  Gain=-1
  Mux1 : Mux  Inputs=3
  Product{2..6} (5 alike) : Product  RndMeth=Zero
  Terminator4 : Terminator
  Trigonometric Function1 : Trigonometry  Operator=cos
  Trigonometric Function2 : Trigonometry
  Trigonometric Function3 : Trigonometry  Operator=cos
  Trigonometric Function4 : Trigonometry
  Weight Force : Constant  Value=nfs.weight
  Weight Moment : Constant  Value=[0 0 0]'
  Force : Outport  Unit=N  PortDimensions=[3,1]
  Moment : Outport  Port=2  Unit=N*m  PortDimensions=[3,1]
  wires:
  Mux1/1 -> Force/1
  Product6/1 -> Mux1/3
  Product3/1 -> Mux1/2
  Product2/1 -> Mux1/1
  Product5/1 -> Product6/2
  Product4/1 -> Product3/1
  Trigonometric Function1/1 -> Product5/2
  Trigonometric Function4/1 -> Product4/1
  Trigonometric Function3/1 -> Product5/1, Product4/2
  Trigonometric Function2/1 -> Gain1/1
  Weight Force/1 -> Product6/1, Product3/2, Product2/2
  Gain1/1 -> Product2/1
  Demux/3 -> Terminator4/1
  Attitute/1 -> Demux/1
  Demux/2 -> Trigonometric Function3/1, Trigonometric Function2/1
  Demux/1 -> Trigonometric Function1/1, Trigonometric Function4/1
  Weight Moment/1 -> Moment/1

== system AFDNFSmodelMPA/OnBoardComputer/Control System/BusCreator ==
  " " : Inport
  Bus Creator : BusCreator  Inputs=4
  Demux2 : Demux
  "  " : Outport
  wires:
  " "/1 -> Demux2/1
  Bus Creator/1 -> "  "/1
  Demux2/1 -> Bus Creator/1  "delta_e"
  Demux2/2 -> Bus Creator/2  "delta_f"
  Demux2/4 -> Bus Creator/4  "delta_r"
  Demux2/3 -> Bus Creator/3  "delta_a"

== system AFDNFSmodelMPA/OnBoardComputer/Control System/Full-State Feedback Servo ==
  States : Inport
  Gain : Gain  Gain=-K_long  Multiplication=Matrix(K*u) (u vector)
  Gain1 : Gain  Gain=-K_lat  Multiplication=Matrix(K*u) (u vector)
  Selector1 : Selector  InputPortWidth=9  IndexOptions=Index vector (dialog)  Indices=[5:9]  OutputSizes=1
  Selector3 : Selector  InputPortWidth=9  IndexOptions=Index vector (dialog)  Indices=[1:4]  OutputSizes=1
  Longitudinal Control : Outport
  Lateral-Directional Control : Outport  Port=2
  wires:
  States/1 -> Selector3/1, Selector1/1
  Selector3/1 -> Gain/1  "Longitudinal"
  Selector1/1 -> Gain1/1  "Lateral-Directional"
  Gain/1 -> Longitudinal Control/1
  Gain1/1 -> Lateral-Directional Control/1

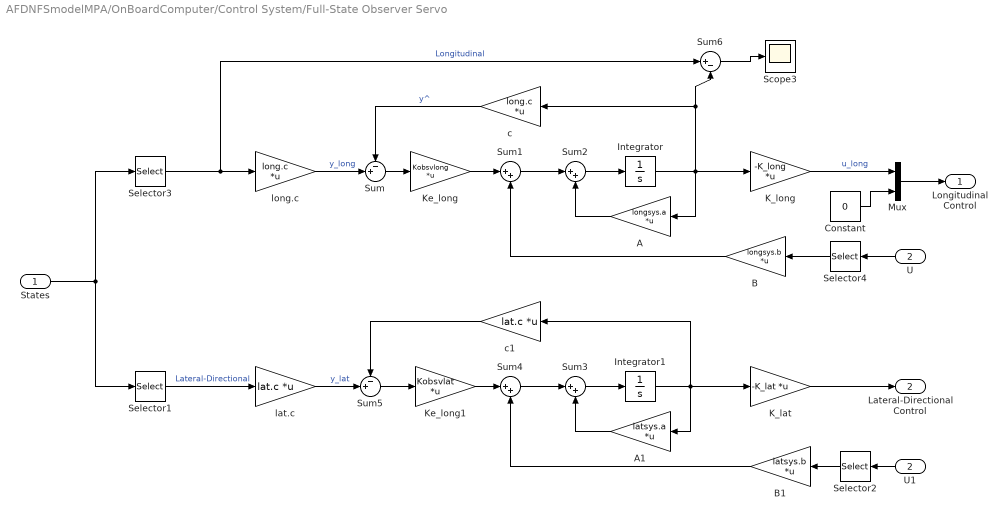
== system AFDNFSmodelMPA/OnBoardComputer/Control System/Full-State Observer Servo ==
  States : Inport  PortDimensions=[9,1]
  U : Inport  Port=2  PortDimensions=[4,1]
  A : Gain  Gain=longsys.a  Multiplication=Matrix(K*u)
  A1 : Gain  Gain=latsys.a  Multiplication=Matrix(K*u)
  B : Gain  Gain=longsys.b  Multiplication=Matrix(K*u)
  B1 : Gain  Gain=latsys.b  Multiplication=Matrix(K*u)
  Constant : Constant  Value=0
  Integrator : Integrator
  Integrator1 : Integrator
  K_lat : Gain  Gain=-K_lat  Multiplication=Matrix(K*u)
  K_long : Gain  Gain=-K_long  Multiplication=Matrix(K*u)
  Ke_long : Gain  Gain=Kobsvlong  Multiplication=Matrix(K*u)
  Ke_long1 : Gain  Gain=Kobsvlat  Multiplication=Matrix(K*u)
  Mux : Mux  Inputs=2
  Scope3 : Scope
  Selector1 : Selector  InputPortWidth=9  IndexOptions=Index vector (dialog)  Indices=[5:9]  OutputSizes=1
  Selector2 : Selector  InputPortWidth=4  IndexOptions=Index vector (dialog)  Indices=[3:4]  OutputSizes=1
  Selector3 : Selector  InputPortWidth=9  IndexOptions=Index vector (dialog)  Indices=[1:4]  OutputSizes=1
  Selector4 : Selector  InputPortWidth=4  IndexOptions=Index vector (dialog)  Indices=[1]  OutputSizes=1
  Sum : Sum  Inputs=-+|
  Sum{1..4} (4 alike) : Sum  Inputs=|++
  Sum5 : Sum  Inputs=-+|
  Sum6 : Sum  Inputs=|+-
  U1 : InportShadow  Port=2  PortDimensions=[4,1]
  c : Gain  Gain=long.c  Multiplication=Matrix(K*u)
  c1 : Gain  Gain=lat.c  Multiplication=Matrix(K*u)
  lat.c : Gain  Gain=lat.c  Multiplication=Matrix(K*u)
  long.c : Gain  Gain=long.c  Multiplication=Matrix(K*u)
  Longitudinal Control : Outport
  Lateral-Directional Control : Outport  Port=2
  wires:
  K_lat/1 -> Lateral-Directional Control/1
  Selector1/1 -> lat.c/1  "Lateral-Directional"
  Selector3/1 -> long.c/1, Sum6/1  "Longitudinal"
  States/1 -> Selector1/1, Selector3/1
  Sum/1 -> Ke_long/1
  Ke_long/1 -> Sum1/1
  B/1 -> Sum1/2
  Sum1/1 -> Sum2/1
  Sum2/1 -> Integrator/1
  Integrator/1 -> A/1, K_long/1, c/1, Sum6/2
  A/1 -> Sum2/2
  long.c/1 -> Sum/2  "y_long"
  c/1 -> Sum/1  "y^"
  Integrator1/1 -> K_lat/1, A1/1, c1/1
  lat.c/1 -> Sum5/2  "y_lat"
  Sum5/1 -> Ke_long1/1
  Ke_long1/1 -> Sum4/1
  Sum4/1 -> Sum3/1
  Sum3/1 -> Integrator1/1
  A1/1 -> Sum3/2
  B1/1 -> Sum4/2
  c1/1 -> Sum5/1
  Sum6/1 -> Scope3/1
  U/1 -> Selector4/1
  U1/1 -> Selector2/1
  Selector4/1 -> B/1
  Selector2/1 -> B1/1
  Mux/1 -> Longitudinal Control/1
  K_long/1 -> Mux/1  "u_long"
  Constant/1 -> Mux/2

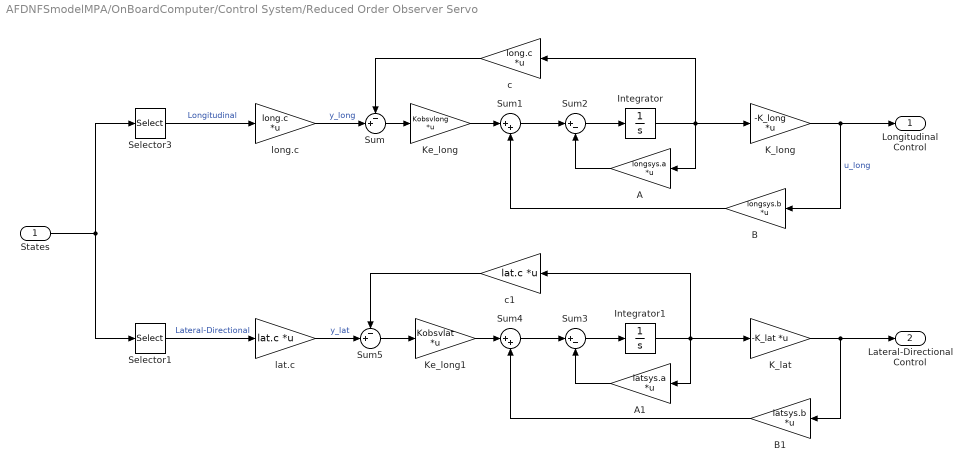
== system AFDNFSmodelMPA/OnBoardComputer/Control System/Reduced Order Observer Servo ==
  States : Inport  PortDimensions=[9,1]
  A : Gain  Gain=longsys.a  Multiplication=Matrix(K*u)
  A1 : Gain  Gain=latsys.a  Multiplication=Matrix(K*u)
  B : Gain  Gain=longsys.b  Multiplication=Matrix(K*u)
  B1 : Gain  Gain=latsys.b  Multiplication=Matrix(K*u)
  Integrator : Integrator
  Integrator1 : Integrator
  K_lat : Gain  Gain=-K_lat  Multiplication=Matrix(K*u)
  K_long : Gain  Gain=-K_long  Multiplication=Matrix(K*u)
  Ke_long : Gain  Gain=Kobsvlong  Multiplication=Matrix(K*u)
  Ke_long1 : Gain  Gain=Kobsvlat  Multiplication=Matrix(K*u)
  Selector1 : Selector  InputPortWidth=9  IndexOptions=Index vector (dialog)  Indices=[5:9]  OutputSizes=1
  Selector3 : Selector  InputPortWidth=9  IndexOptions=Index vector (dialog)  Indices=[1:4]  OutputSizes=1
  Sum : Sum  Inputs=-+|
  Sum1 : Sum  Inputs=|++
  Sum2 : Sum  Inputs=|+-
  Sum3 : Sum  Inputs=|+-
  Sum4 : Sum  Inputs=|++
  Sum5 : Sum  Inputs=-+|
  c : Gain  Gain=long.c  Multiplication=Matrix(K*u)
  c1 : Gain  Gain=lat.c  Multiplication=Matrix(K*u)
  lat.c : Gain  Gain=lat.c  Multiplication=Matrix(K*u)
  long.c : Gain  Gain=long.c  Multiplication=Matrix(K*u)
  Longitudinal Control : Outport
  Lateral-Directional Control : Outport  Port=2
  wires:
  c1/1 -> Sum5/1
  B1/1 -> Sum4/2
  A1/1 -> Sum3/2
  Sum3/1 -> Integrator1/1
  Sum4/1 -> Sum3/1
  Ke_long1/1 -> Sum4/1
  Sum5/1 -> Ke_long1/1
  lat.c/1 -> Sum5/2  "y_lat"
  Integrator1/1 -> c1/1, A1/1, K_lat/1
  c/1 -> Sum/1
  long.c/1 -> Sum/2  "y_long"
  A/1 -> Sum2/2
  Integrator/1 -> c/1, K_long/1, A/1
  Sum2/1 -> Integrator/1
  Sum1/1 -> Sum2/1
  B/1 -> Sum1/2
  Ke_long/1 -> Sum1/1
  Sum/1 -> Ke_long/1
  States/1 -> Selector3/1, Selector1/1
  Selector3/1 -> long.c/1  "Longitudinal"
  Selector1/1 -> lat.c/1  "Lateral-Directional"
  K_long/1 -> B/1, Longitudinal Control/1  "u_long"
  K_lat/1 -> B1/1, Lateral-Directional Control/1

== system AFDNFSmodelMPA/OnBoardComputer/Control System/Trim ==
  Bus Creator : BusCreator  Inputs=4
  Constant2 : Constant  Value=nfs.trim.delta_e
  Constant3 : Constant  Value=0
  Constant4 : Constant  Value=0
  Constant5 : Constant  Value=0
  Doublet Generated Signal : Subsystem
  Manual Switch : ManualSwitch  CurrentSetting=0
  Manual Switch1 : ManualSwitch  CurrentSetting=0
  Scope : Scope
  Triangular signal span 10 sec : Subsystem
  Out1 : Outport
  wires:
  Bus Creator/1 -> Manual Switch/2
  Doublet Generated Signal/1(Doublet Out) -> Manual Switch1/1
  Triangular signal span 10 sec/1(Tri) -> Manual Switch1/2
  Manual Switch1/1 -> Scope/1, Manual Switch/1
  Manual Switch/1 -> Out1/1
  Constant2/1 -> Bus Creator/1  "delta_e"
  Constant3/1 -> Bus Creator/2  "delta_f"
  Constant5/1 -> Bus Creator/4  "delta_r"
  Constant4/1 -> Bus Creator/3  "delta_a"

== system AFDNFSmodelMPA/Nonlinear Flight Simulator/6DoF Nonlinear Flight Equations of Motion (Rigid Body)/AngularAcceleration(Omegadot)/Cross Product ==
  A : Inport
  B : Inport  Port=2
  "A " : InportShadow
  "B " : InportShadow  Port=2
  Subsystem2 : Subsystem
  Subsystem3 : Subsystem
  Sum : Sum  Inputs=+|-  SaturateOnIntegerOverflow=on  InputSameDT=on  OutDataTypeStr=Inherit: Same as first input
  C : Outport
  wires:
  Subsystem3/1(Out2) -> Sum/2
  Subsystem2/1(Out1) -> Sum/1
  A/1 -> Subsystem2/1(A)
  B/1 -> Subsystem2/2(B)
  Sum/1 -> C/1
  "A "/1 -> Subsystem3/1(A)
  "B "/1 -> Subsystem3/2(B)

== system AFDNFSmodelMPA/Nonlinear Flight Simulator/6DoF Nonlinear Flight Equations of Motion (Rigid Body)/Euler angles & Direction Cosine/Euler angles Calculation ==
  Angular Velocities : Inport  PortDimensions=[3,1]
  Euler Angles : Inport  Port=2
  Mux1 : Mux  Inputs=[3 3 3]
  Mux2 : Mux  Inputs=3
  phidot : Fcn  Expr=u[1]+(u[2]*u[4]+u[3]*u[7])*(u[5]/u[8])
  psidot : Fcn  Expr=(u[2]*u[4]+u[3]*u[7])/u[8]
  sincos : Trigonometry  Operator=sincos
  thetadot : Fcn  Expr=u[2]*u[7]-u[3]*u[4]
  Euler Rates : Outport  PortDimensions=[3,1]  InitialOutput=0
  wires:
  sincos/2 -> Mux1/3
  sincos/1 -> Mux1/2
  Mux2/1 -> Euler Rates/1
  phidot/1 -> Mux2/1
  thetadot/1 -> Mux2/2
  psidot/1 -> Mux2/3
  Euler Angles/1 -> sincos/1
  Angular Velocities/1 -> Mux1/1
  Mux1/1 -> psidot/1, phidot/1, thetadot/1

== system AFDNFSmodelMPA/Nonlinear Flight Simulator/6DoF Nonlinear Flight Equations of Motion (Rigid Body)/Euler angles & Direction Cosine/If Action Subsystem ==
  Simulation Termination : Inport
  Action Port : ActionPort  ActionType=then
  Stop Simulation : Stop
  wires:
  Simulation Termination/1 -> Stop Simulation/1

== system AFDNFSmodelMPA/Nonlinear Flight Simulator/6DoF Nonlinear Flight Equations of Motion (Rigid Body)/Euler angles & Direction Cosine/Rotation Angles to DCM ==
  "[R1,R2,R3]" : Inport  PortDimensions=3
  Create 3x3 Matrix : aerolibutil/Create 3x3 Matrix
  Fcn11 : Fcn  Expr=u(5)*u(4)
  Fcn12 : Fcn  Expr=u(5)*u(1)
  Fcn13 : Fcn  Expr=-u(2)
  Fcn21 : Fcn  Expr=u(3)*u(2)*u(4) - u(6)*u(1)
  Fcn22 : Fcn  Expr=u(3)*u(2)*u(1) + u(6)*u(4)
  Fcn23 : Fcn  Expr=u(3)*u(5)
  Fcn31 : Fcn  Expr=u(6)*u(2)*u(4) + u(3)*u(1)
  Fcn32 : Fcn  Expr=u(6)*u(2)*u(1) - u(3)*u(4)
  Fcn33 : Fcn  Expr=u(6)*u(5)
  Mux : Mux  Inputs=2
  sincos1 : Trigonometry  Operator=sincos
  DCM : Outport  PortDimensions=[3,3]
  wires:
  "[R1,R2,R3]"/1 -> sincos1/1
  Create 3x3 Matrix/1 -> DCM/1
  sincos1/1 -> Mux/1
  sincos1/2 -> Mux/2
  Mux/1 -> Fcn32/1, Fcn33/1, Fcn31/1, Fcn23/1, Fcn22/1, Fcn11/1, Fcn12/1, Fcn13/1, Fcn21/1
  Fcn11/1 -> Create 3x3 Matrix/1
  Fcn12/1 -> Create 3x3 Matrix/2
  Fcn13/1 -> Create 3x3 Matrix/3
  Fcn21/1 -> Create 3x3 Matrix/4
  Fcn31/1 -> Create 3x3 Matrix/7
  Fcn22/1 -> Create 3x3 Matrix/5
  Fcn23/1 -> Create 3x3 Matrix/6
  Fcn32/1 -> Create 3x3 Matrix/8
  Fcn33/1 -> Create 3x3 Matrix/9

== system AFDNFSmodelMPA/Nonlinear Flight Simulator/6DoF Nonlinear Flight Equations of Motion (Rigid Body)/Euler angles & Direction Cosine/Transform from Body to Inertial axes ==
  Transformation Matrix : Inport
  Position Vector : Inport  Port=2
  Product : Product  Multiplication=Matrix(*)  SaturateOnIntegerOverflow=on  InputSameDT=on  OutDataTypeStr=Inherit: Same as first input
  Reshape1 : Reshape  OutputDimensionality=Column vector (2-D)
  Reshape2 : Reshape
  Ve : Outport
  wires:
  Reshape2/1 -> Ve/1
  Reshape1/1 -> Product/2
  Position Vector/1 -> Reshape1/1
  Transformation Matrix/1 -> Product/1
  Product/1 -> Reshape2/1

== system AFDNFSmodelMPA/Nonlinear Flight Simulator/6DoF Nonlinear Flight Equations of Motion (Rigid Body)/Linear Acceleration(Vdot)/Cross Product ==
  A : Inport
  B : Inport  Port=2
  "A " : InportShadow
  "B " : InportShadow  Port=2
  Subsystem2 : Subsystem
  Subsystem3 : Subsystem
  Sum : Sum  Inputs=+|-  SaturateOnIntegerOverflow=on  InputSameDT=on  OutDataTypeStr=Inherit: Same as first input
  C : Outport
  wires:
  Subsystem3/1(Out2) -> Sum/2
  Subsystem2/1(Out1) -> Sum/1
  A/1 -> Subsystem2/1(A)
  B/1 -> Subsystem2/2(B)
  Sum/1 -> C/1
  "A "/1 -> Subsystem3/1(A)
  "B "/1 -> Subsystem3/2(B)

== system AFDNFSmodelMPA/Nonlinear Flight Simulator/Forces&Moments/Aero Attributes/Dynamic Pressure Calc ==
  Air Density : Inport  PortDimensions=1
  Linear Velocity (Body) : Inport  Port=2  PortDimensions=[3 1]
  0.5*rh : Product  SaturateOnIntegerOverflow=on  InputSameDT=on  OutDataTypeStr=Inherit: Same as first input
  Dot Product : DotProduct  InputSameDT=on  OutDataTypeStr=Inherit: Inherit via internal rule
  Gain : Gain  Gain=0.5  SaturateOnIntegerOverflow=on  OutDataTypeStr=Inherit: Same as input  ParamDataTypeStr=Inherit: Same as input
  V^2 : Abs
  Dynamic Pressure : Outport
  wires:
  Dot Product/1 -> V^2/1
  Linear Velocity (Body)/1 -> Dot Product/2, Dot Product/1
  Air Density/1 -> Gain/1
  V^2/1 -> 0.5*rh/1
  Gain/1 -> 0.5*rh/2
  0.5*rh/1 -> Dynamic Pressure/1

== system AFDNFSmodelMPA/Nonlinear Flight Simulator/Forces&Moments/Aero Attributes/Subsystem ==
  Height : Inport
  "(T/T0)^(g/LR) " : Math  Operator=pow  SaturateOnIntegerOverflow=on
  1/T0 : Gain  Gain=1/288.15  SaturateOnIntegerOverflow=on  OutDataTypeStr=Inherit: Same as input  ParamDataTypeStr=Inherit: Same as input
  Altitude of Troposphere : Constant  Value=11000  OutDataTypeStr=Inherit: Inherit via back propagation
  Lapse Rate : Gain  Gain=0.0065  SaturateOnIntegerOverflow=on  OutDataTypeStr=Inherit: Same as input  ParamDataTypeStr=Inherit: Same as input
  Limit  altitude  to Stratosphere : Saturate  UpperLimit=0  LowerLimit=11000-20000
  Limit  altitude  to troposhere : Saturate  UpperLimit=11000  LowerLimit=0
  Product : Product  Inputs=*/  SaturateOnIntegerOverflow=on  InputSameDT=on  OutDataTypeStr=Inherit: Same as first input
  Product1 : Product  Inputs=/*  SaturateOnIntegerOverflow=on  InputSameDT=on  OutDataTypeStr=Inherit: Same as first input
  Product3 : Product  SaturateOnIntegerOverflow=on  InputSameDT=on  OutDataTypeStr=Inherit: Same as first input
  Sea Level  Temperature : Constant  Value=288.15  OutDataTypeStr=Inherit: Inherit via back propagation
  Stratosphere Model : Math  SaturateOnIntegerOverflow=on
  Sum : Sum  Inputs=+-  SaturateOnIntegerOverflow=on  InputSameDT=on  OutDataTypeStr=Inherit: Same as first input
  Sum1 : Sum  Inputs=+-  SaturateOnIntegerOverflow=on  InputSameDT=on  OutDataTypeStr=Inherit: Same as first input
  a : Sqrt  AlgorithmType=Newton-Raphson  SaturateOnIntegerOverflow=on
  g/(L*R) : Constant  Value=9.80665/(0.0065*287.0531)  OutDataTypeStr=Inherit: Inherit via back propagation
  g/R : Gain  Gain=9.80665/287.0531  SaturateOnIntegerOverflow=on  OutDataTypeStr=Inherit: Same as input  ParamDataTypeStr=Inherit: Same as input
  gamma*R : Gain  Gain=1.4*287.0531  SaturateOnIntegerOverflow=on  OutDataTypeStr=Inherit: Same as input  ParamDataTypeStr=Inherit: Same as input
  rho0 : Gain  Gain=1.225  SaturateOnIntegerOverflow=on  OutDataTypeStr=Inherit: Same as input  ParamDataTypeStr=Inherit: Same as input
  Speed of Sound : Outport  PortDimensions=1
  Air Density : Outport  Port=2  PortDimensions=1
  wires:
  g/(L*R)/1 -> "(T/T0)^(g/LR) "/2
  Height/1 -> Limit  altitude  to troposhere/1, Sum/2
  Limit  altitude  to troposhere/1 -> Lapse Rate/1
  Product/1 -> rho0/1
  "(T/T0)^(g/LR) "/1 -> Product/1
  1/T0/1 -> "(T/T0)^(g/LR) "/1, Product/2
  gamma*R/1 -> a/1
  a/1 -> Speed of Sound/1
  Sum1/1 -> gamma*R/1, 1/T0/1, Product1/1
  Lapse Rate/1 -> Sum1/2
  Sea Level  Temperature/1 -> Sum1/1
  rho0/1 -> Product3/1
  Product3/1 -> Air Density/1
  Stratosphere Model/1 -> Product3/2
  g/R/1 -> Product1/2
  Product1/1 -> Stratosphere Model/1
  Altitude of Troposphere/1 -> Sum/1
  Sum/1 -> Limit  altitude  to Stratosphere/1
  Limit  altitude  to Stratosphere/1 -> g/R/1
